simulink model "turbine_th"  (R2018b)
settings: Solver=VariableStepAuto  StartTime=0.0  StopTime=0  RelTol=1e-3
libraries: turbine_ul x1
settings Model: Creator=mcobb  LastModifiedBy=mcobb

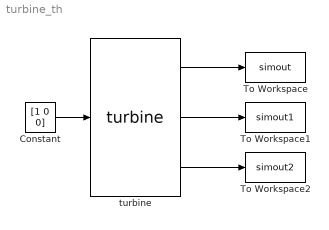
== system turbine_th ==
  Constant : Constant  Value=[1 0 0]
  To Workspace : ToWorkspace  VariableName=simout  SaveFormat=Timeseries  SampleTime=-1
  To Workspace1 : ToWorkspace  VariableName=simout1  SaveFormat=Timeseries  SampleTime=-1
  To Workspace2 : ToWorkspace  VariableName=simout2  SaveFormat=Timeseries  SampleTime=-1
  turbine : turbine_ul/turbine  diam=d  Cp=Cp  Cd=Cd  rho=rho  rTurb=turbPosVec
  wires:
  Constant/1 -> turbine/1
  turbine/1 -> To Workspace/1
  turbine/2 -> To Workspace1/1
  turbine/3 -> To Workspace2/1
